simulink model "planta"  (R2021a)
settings: Solver=FixedStepAuto  StartTime=0.0  StopTime=10.0  RelTol=1e-3  EnableMultiTasking=on
settings Model: Creator=exupe  LastModifiedBy=lucas
settings SolverCC: AlgebraicLoopSolver=TrustRegion
settings DataIOCC: ReturnWorkspaceOutputs=off
settings OptimizationCC: LifeSpan=inf
settings DebuggingCC: SFUnexpectedBacktrackingDiag=warning  SFNoUnconditionalDefaultTransitionDiag=warning  SFMachineParentedDataDiag=warning  ArithmeticOperatorsInVariantConditions=warning
settings SFSimCC: SimUseLocalCustomCode=off  CustomCodeUndefinedFunction=UseInterfaceOnly
settings RTWCC: RTWUseLocalCustomCode=off
settings CodeAppCC: StateflowObjectComments=on
settings GRTTargetCC: TargetLangStandard=C89/C90 (ANSI)
settings ConfigComp: CovMetricSettings=dw  CovSaveCumulativeToWorkspaceVar=on  CovSaveSingleToWorkspaceVar=on  CovExternalEMLEnable=off

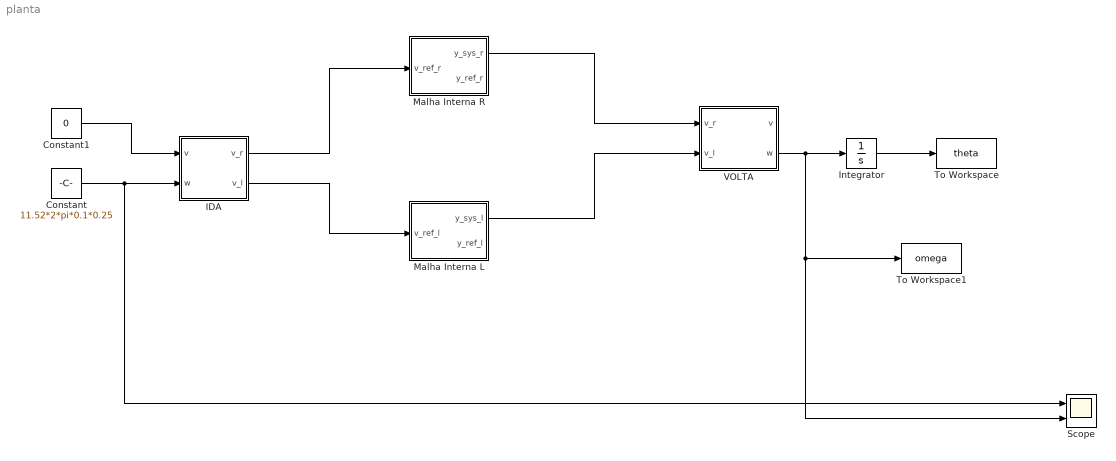
== system planta ==
  Constant : Constant  Value=11.52*2*pi*0.1*0.25
  Constant1 : Constant  Value=0
  IDA : Subsystem
  Integrator : Integrator
  Malha Interna L : Subsystem
  Malha Interna R : Subsystem
  Scope : Scope  NumInputPorts=2
  To Workspace : ToWorkspace  VariableName=theta  SaveFormat=Timeseries  SampleTime=-1
  To Workspace1 : ToWorkspace  VariableName=omega  SampleTime=-1
  VOLTA : Subsystem
  wires:
  IDA/1(v_r) -> Malha Interna R/1(v_ref_r)
  IDA/2(v_l) -> Malha Interna L/1(v_ref_l)
  Malha Interna L/1(y_sys_l) -> VOLTA/2(v_l)
  Malha Interna R/1(y_sys_r) -> VOLTA/1(v_r)
  VOLTA/2(w) -> To Workspace1/1, Scope/2, Integrator/1
  Integrator/1 -> To Workspace/1
  Constant/1 -> Scope/1, IDA/2(w)
  Constant1/1 -> IDA/1(v)

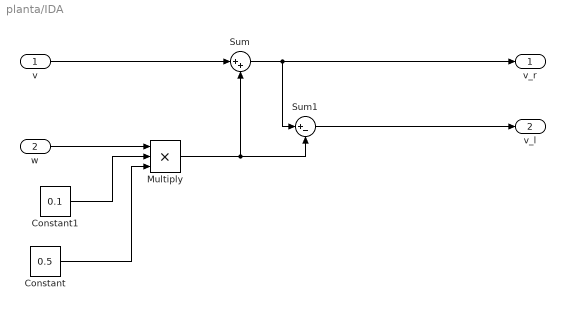
== system planta/IDA ==
  v : Inport
  w : Inport  Port=2
  Constant : Constant  Value=0.5
  Constant1 : Constant  Value=0.1
  Multiply : Product  Inputs=3
  Sum : Sum  Inputs=|++
  Sum1 : Sum  Inputs=|+-
  v_r : Outport  VectorParamsAs1DForOutWhenUnconnected=off
  v_l : Outport  Port=2  VectorParamsAs1DForOutWhenUnconnected=off
  wires:
  Multiply/1 -> Sum1/2, Sum/2
  Sum1/1 -> v_l/1
  Constant1/1 -> Multiply/2
  v/1 -> Sum/1
  w/1 -> Multiply/1
  Sum/1 -> v_r/1, Sum1/1
  Constant/1 -> Multiply/3

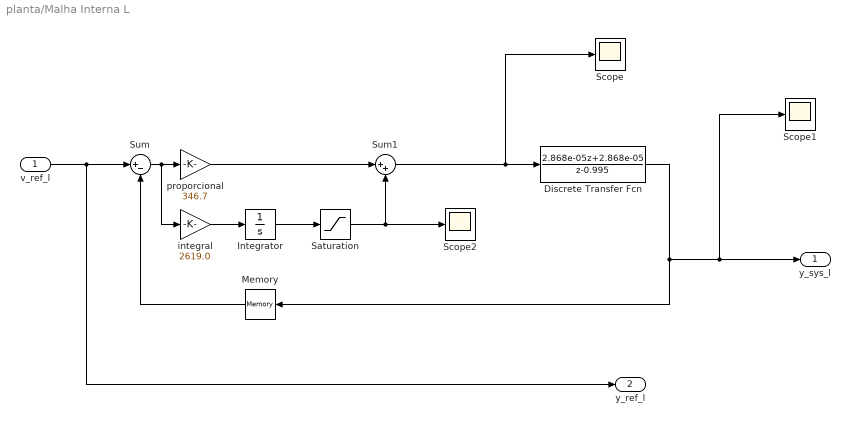
== system planta/Malha Interna L ==
  v_ref_l : Inport
  Discrete Transfer Fcn : DiscreteTransferFcn  Numerator=[2.868e-05 2.868e-05]  Denominator=[1 -0.995]  SampleTime=0.001
  Integrator : Integrator
  Memory : Memory
  Saturation : Saturate  UpperLimit=4095  LowerLimit=0
  Scope : Scope
  Scope1 : Scope
  Scope2 : Scope
  Sum : Sum  Inputs=|+-
  Sum1 : Sum  Inputs=|++
  integral : Gain  Gain=2619.0
  proporcional : Gain  Gain=346.7
  y_sys_l : Outport  VectorParamsAs1DForOutWhenUnconnected=off
  "y_ref_l " : Outport  Port=2  VectorParamsAs1DForOutWhenUnconnected=off
  wires:
  Memory/1 -> Sum/2
  Saturation/1 -> Scope2/1, Sum1/2
  proporcional/1 -> Sum1/1
  v_ref_l/1 -> "y_ref_l "/1, Sum/1
  Sum1/1 -> Scope/1, Discrete Transfer Fcn/1
  Discrete Transfer Fcn/1 -> Memory/1, y_sys_l/1, Scope1/1
  integral/1 -> Integrator/1
  Sum/1 -> integral/1, proporcional/1
  Integrator/1 -> Saturation/1

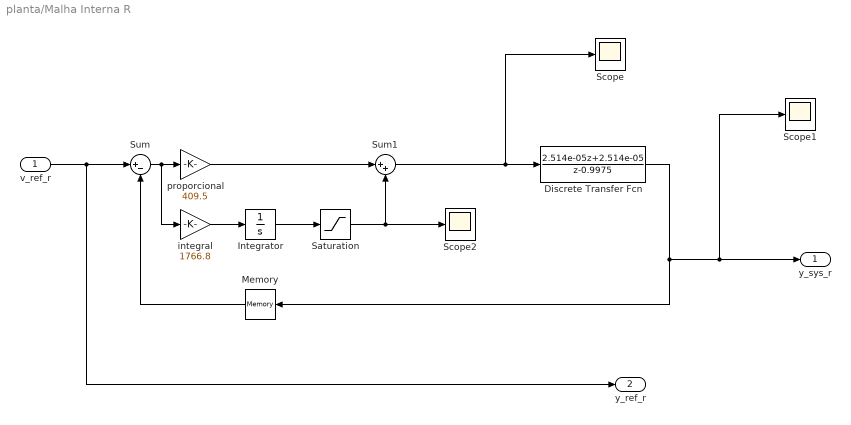
== system planta/Malha Interna R ==
  v_ref_r : Inport
  Discrete Transfer Fcn : DiscreteTransferFcn  Numerator=[2.514e-05 2.514e-05]  Denominator=[1 -0.9975]  SampleTime=0.001
  Integrator : Integrator
  Memory : Memory
  Saturation : Saturate  UpperLimit=4095  LowerLimit=0
  Scope : Scope
  Scope1 : Scope
  Scope2 : Scope
  Sum : Sum  Inputs=|+-
  Sum1 : Sum  Inputs=|++
  integral : Gain  Gain=1766.8
  proporcional : Gain  Gain=409.5
  y_sys_r : Outport  VectorParamsAs1DForOutWhenUnconnected=off
  "y_ref_r " : Outport  Port=2  VectorParamsAs1DForOutWhenUnconnected=off
  wires:
  Memory/1 -> Sum/2
  Saturation/1 -> Scope2/1, Sum1/2
  proporcional/1 -> Sum1/1
  v_ref_r/1 -> "y_ref_r "/1, Sum/1
  Sum1/1 -> Scope/1, Discrete Transfer Fcn/1
  Discrete Transfer Fcn/1 -> Memory/1, y_sys_r/1, Scope1/1
  integral/1 -> Integrator/1
  Sum/1 -> integral/1, proporcional/1
  Integrator/1 -> Saturation/1

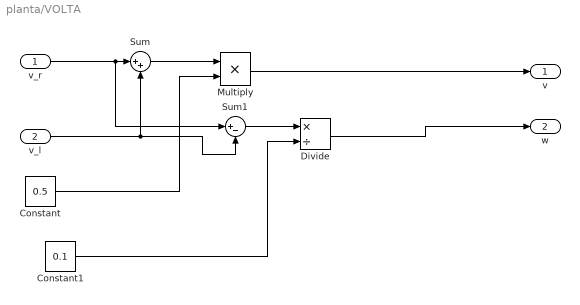
== system planta/VOLTA ==
  v_r : Inport
  v_l : Inport  Port=2
  Constant : Constant  Value=0.5
  Constant1 : Constant  Value=0.1
  Divide : Product  Inputs=*/
  Multiply : Product
  Sum : Sum  Inputs=|++
  Sum1 : Sum  Inputs=|+-
  v : Outport  VectorParamsAs1DForOutWhenUnconnected=off
  w : Outport  Port=2  VectorParamsAs1DForOutWhenUnconnected=off
  wires:
  Sum/1 -> Multiply/1
  v_l/1 -> Sum1/2, Sum/2
  Sum1/1 -> Divide/1
  v_r/1 -> Sum1/1, Sum/1
  Constant1/1 -> Divide/2
  Multiply/1 -> v/1
  Divide/1 -> w/1
  Constant/1 -> Multiply/2
